simulink model "Linear_EHA_Model"  (R2018a)
settings: Solver=VariableStepAuto  StartTime=0.0  StopTime=5  RelTol=1e-3
undefined symbols (not defined in the file): K_HA, Kv, L, wn, zeta
settings Model: Creator=UFUK  LastModifiedBy=UFUK

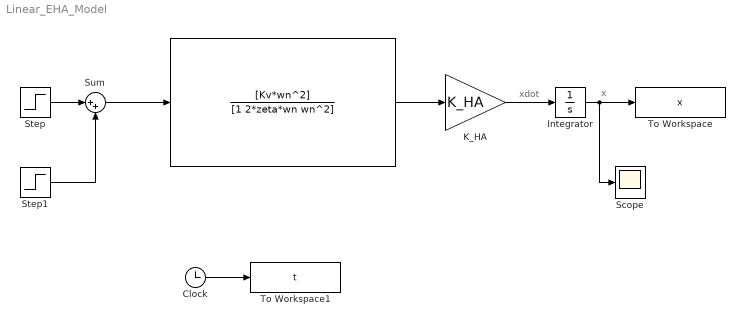
== system Linear_EHA_Model ==
  note: xdot
  note: x
  " " : TransferFcn  Numerator=[Kv*wn^2]  Denominator=[1 2*zeta*wn wn^2]
  " K_HA" : Gain  Gain=K_HA
  Clock : Clock
  Integrator : Integrator  InitialCondition=L/2
  Scope : Scope
  Step : Step  Time=0.5  After=10  SampleTime=0
  Step1 : Step  After=-10  SampleTime=0
  Sum : Sum  Inputs=|++
  To Workspace : ToWorkspace  VariableName=x  SaveFormat=Timeseries  SampleTime=-1
  To Workspace1 : ToWorkspace  VariableName=t  SaveFormat=Timeseries  SampleTime=-1
  wires:
  Step/1 -> Sum/1
  " K_HA"/1 -> Integrator/1
  " "/1 -> " K_HA"/1
  Sum/1 -> " "/1
  Step1/1 -> Sum/2
  Clock/1 -> To Workspace1/1
  Integrator/1 -> Scope/1, To Workspace/1
